simulink model "HANcoder_E407_TTA_Template_DS_V52"  (R2023a)
settings: Solver=FixedStepDiscrete  StartTime=0.0  StopTime=1  FixedStep=0.01  RelTol=1e-3
PreLoadFcn:
  | librarySetup
  | eval([bdroot,'_startup']) %Calling [modelName]_startup.m
values from neighbouring files (symbols this model uses):
  basic_cycle_duration_bc0 = TM_Reset_Board   + COMP_duration    (= 372)    [HANcoder_E407_TTA_Template_DS_V1_startup.m]    (also in HANcoder_E407_TTA_Template_DS_V2_startup.m; HANcoder_E407_TTA_Template_DS_V52_startup.m; HANcoder_E407_TTA_Template_DS_V5_startup.m; HANcoder_E407_TTA_Template_DS_V6_startup.m = 532)
  basic_cycle_duration_bc1 = basic_cycle_duration_bc0    (= 372)    [HANcoder_E407_TTA_Template_DS_V1_startup.m]    (also in HANcoder_E407_TTA_Template_DS_V2_startup.m; HANcoder_E407_TTA_Template_DS_V52_startup.m; HANcoder_E407_TTA_Template_DS_V5_startup.m; HANcoder_E407_TTA_Template_DS_V6_startup.m = 532)
  basic_cycle_duration_bc2 = basic_cycle_duration_bc0    (= 372)    [HANcoder_E407_TTA_Template_DS_V1_startup.m]    (also in HANcoder_E407_TTA_Template_DS_V2_startup.m; HANcoder_E407_TTA_Template_DS_V52_startup.m; HANcoder_E407_TTA_Template_DS_V5_startup.m; HANcoder_E407_TTA_Template_DS_V6_startup.m = 532)
  comm_delay_estimation1 = round(comm_delay_measured1*hardware_granularity/frequency_IRQ)    [HANcoder_E407_TTA_Template_DS_V1_startup.m]    (also in HANcoder_E407_TTA_Template_DS_V2_startup.m; HANcoder_E407_TTA_Template_DS_V52_startup.m; HANcoder_E407_TTA_Template_DS_V5_startup.m; HANcoder_E407_TTA_Template_DS_V6_startup.m)
  comm_delay_estimation2 = round(comm_delay_measured2*hardware_granularity/frequency_IRQ)    [HANcoder_E407_TTA_Template_DS_V1_startup.m]    (also in HANcoder_E407_TTA_Template_DS_V2_startup.m; HANcoder_E407_TTA_Template_DS_V52_startup.m; HANcoder_E407_TTA_Template_DS_V5_startup.m; HANcoder_E407_TTA_Template_DS_V6_startup.m)
  COMM_Period = 80    [HANcoder_E407_TTA_Template_DS_V1_startup.m]    (also in HANcoder_E407_TTA_Template_DS_V2_startup.m; HANcoder_E407_TTA_Template_DS_V52_startup.m; HANcoder_E407_TTA_Template_DS_V5_startup.m; HANcoder_E407_TTA_Template_DS_V6_startup.m = 120)
  COMM_Phase1 = Simulink.Parameter    [HANcoder_E407_TTA_Template_DS_V1_startup.m]    (also in HANcoder_E407_TTA_Template_DS_V2_startup.m; HANcoder_E407_TTA_Template_DS_V52_startup.m; HANcoder_E407_TTA_Template_DS_V5_startup.m; HANcoder_E407_TTA_Template_DS_V6_startup.m)
  COMM_Phase2 = Simulink.Parameter    [HANcoder_E407_TTA_Template_DS_V1_startup.m]    (also in HANcoder_E407_TTA_Template_DS_V2_startup.m; HANcoder_E407_TTA_Template_DS_V52_startup.m; HANcoder_E407_TTA_Template_DS_V5_startup.m; HANcoder_E407_TTA_Template_DS_V6_startup.m)
  COMM_Phase_init1 = Simulink.Parameter    [HANcoder_E407_TTA_Template_DS_V1_startup.m]    (also in HANcoder_E407_TTA_Template_DS_V2_startup.m; HANcoder_E407_TTA_Template_DS_V52_startup.m; HANcoder_E407_TTA_Template_DS_V5_startup.m; HANcoder_E407_TTA_Template_DS_V6_startup.m)
  COMM_Phase_init2 = Simulink.Parameter    [HANcoder_E407_TTA_Template_DS_V1_startup.m]    (also in HANcoder_E407_TTA_Template_DS_V2_startup.m; HANcoder_E407_TTA_Template_DS_V52_startup.m; HANcoder_E407_TTA_Template_DS_V5_startup.m; HANcoder_E407_TTA_Template_DS_V6_startup.m)
  COMP_duration = 4    [HANcoder_E407_TTA_Template_DS_V1_startup.m]    (also in HANcoder_E407_TTA_Template_DS_V2_startup.m; HANcoder_E407_TTA_Template_DS_V52_startup.m; HANcoder_E407_TTA_Template_DS_V5_startup.m; HANcoder_E407_TTA_Template_DS_V6_startup.m)
  frequency_IRQ = 100    [HANcoder_E407_TTA_Template_DS_V1_startup.m]    (also in HANcoder_E407_TTA_Template_DS_V2_startup.m; HANcoder_E407_TTA_Template_DS_V52_startup.m; HANcoder_E407_TTA_Template_DS_V5_startup.m; HANcoder_E407_TTA_Template_DS_V6_startup.m)
  idle_time_init = basic_cycle_duration_bc0 + basic_cycle_duration_bc1    (= 744)    [HANcoder_E407_TTA_Template_DS_V1_startup.m]    (also in HANcoder_E407_TTA_Template_DS_V2_startup.m; HANcoder_E407_TTA_Template_DS_V52_startup.m = 1116; HANcoder_E407_TTA_Template_DS_V5_startup.m = 1116; HANcoder_E407_TTA_Template_DS_V6_startup.m = 1596)
  L0b = 0.5    [HANcoder_E407_TTA_Template_DS_V52_startup.m]    (also in HANcoder_E407_TTA_Template_DS_V5_startup.m; HANcoder_E407_TTA_Template_DS_V6_startup.m)
  L0f = 5    [HANcoder_E407_TTA_Template_DS_V52_startup.m]    (also in HANcoder_E407_TTA_Template_DS_V5_startup.m; HANcoder_E407_TTA_Template_DS_V6_startup.m)
  L1f = 6    [HANcoder_E407_TTA_Template_DS_V52_startup.m]    (also in HANcoder_E407_TTA_Template_DS_V5_startup.m; HANcoder_E407_TTA_Template_DS_V6_startup.m)
  LA_Clock_Gr = 1    [HANcoder_E407_TTA_Template_DS_V1_startup.m]    (also in HANcoder_E407_TTA_Template_DS_V2_startup.m; HANcoder_E407_TTA_Template_DS_V52_startup.m; HANcoder_E407_TTA_Template_DS_V5_startup.m; HANcoder_E407_TTA_Template_DS_V6_startup.m)
  LA_COMM_dly = 1    [HANcoder_E407_TTA_Template_DS_V1_startup.m]    (also in HANcoder_E407_TTA_Template_DS_V2_startup.m; HANcoder_E407_TTA_Template_DS_V52_startup.m; HANcoder_E407_TTA_Template_DS_V5_startup.m; HANcoder_E407_TTA_Template_DS_V6_startup.m)
  LA_COMM_Err = 1    [HANcoder_E407_TTA_Template_DS_V1_startup.m]    (also in HANcoder_E407_TTA_Template_DS_V2_startup.m; HANcoder_E407_TTA_Template_DS_V52_startup.m; HANcoder_E407_TTA_Template_DS_V5_startup.m; HANcoder_E407_TTA_Template_DS_V6_startup.m)
  LA_E_Desync = 1    [HANcoder_E407_TTA_Template_DS_V1_startup.m]    (also in HANcoder_E407_TTA_Template_DS_V2_startup.m; HANcoder_E407_TTA_Template_DS_V52_startup.m; HANcoder_E407_TTA_Template_DS_V5_startup.m; HANcoder_E407_TTA_Template_DS_V6_startup.m)
  LA_MEX_Flag = 1    [HANcoder_E407_TTA_Template_DS_V1_startup.m]    (also in HANcoder_E407_TTA_Template_DS_V2_startup.m; HANcoder_E407_TTA_Template_DS_V52_startup.m; HANcoder_E407_TTA_Template_DS_V5_startup.m; HANcoder_E407_TTA_Template_DS_V6_startup.m)
  LA_Task_Act = 1    [HANcoder_E407_TTA_Template_DS_V1_startup.m]    (also in HANcoder_E407_TTA_Template_DS_V2_startup.m; HANcoder_E407_TTA_Template_DS_V52_startup.m; HANcoder_E407_TTA_Template_DS_V5_startup.m; HANcoder_E407_TTA_Template_DS_V6_startup.m)
  Master_Role = 1    [HANcoder_E407_TTA_Template_DS_V1_startup.m]    (also in HANcoder_E407_TTA_Template_DS_V2_startup.m; HANcoder_E407_TTA_Template_DS_V52_startup.m; HANcoder_E407_TTA_Template_DS_V5_startup.m; HANcoder_E407_TTA_Template_DS_V6_startup.m)
  matrix_rows = 3    [HANcoder_E407_TTA_Template_DS_V1_startup.m]    (also in HANcoder_E407_TTA_Template_DS_V2_startup.m; HANcoder_E407_TTA_Template_DS_V52_startup.m; HANcoder_E407_TTA_Template_DS_V5_startup.m; HANcoder_E407_TTA_Template_DS_V6_startup.m)
  max_desync = 15    [HANcoder_E407_TTA_Template_DS_V1_startup.m]    (also in HANcoder_E407_TTA_Template_DS_V2_startup.m; HANcoder_E407_TTA_Template_DS_V52_startup.m; HANcoder_E407_TTA_Template_DS_V5_startup.m; HANcoder_E407_TTA_Template_DS_V6_startup.m)
  max_num_msgs_CAN1 = 2^Tx_bit_number-1    (= 7)    [HANcoder_E407_TTA_Template_DS_V1_startup.m]    (also in HANcoder_E407_TTA_Template_DS_V2_startup.m; HANcoder_E407_TTA_Template_DS_V52_startup.m; HANcoder_E407_TTA_Template_DS_V5_startup.m; HANcoder_E407_TTA_Template_DS_V6_startup.m)
  max_num_msgs_CAN2 = max_num_msgs_CAN1    (= 7)    [HANcoder_E407_TTA_Template_DS_V1_startup.m]    (also in HANcoder_E407_TTA_Template_DS_V2_startup.m; HANcoder_E407_TTA_Template_DS_V52_startup.m; HANcoder_E407_TTA_Template_DS_V5_startup.m; HANcoder_E407_TTA_Template_DS_V6_startup.m)
  min_desync = (-1)*max_desync    (= -15)    [HANcoder_E407_TTA_Template_DS_V1_startup.m]    (also in HANcoder_E407_TTA_Template_DS_V2_startup.m; HANcoder_E407_TTA_Template_DS_V52_startup.m; HANcoder_E407_TTA_Template_DS_V5_startup.m; HANcoder_E407_TTA_Template_DS_V6_startup.m)
  PID_derivative = Simulink.Parameter    [HANcoder_E407_TTA_Template_DS_V52_startup.m]    (also in HANcoder_E407_TTA_Template_DS_V6_startup.m)
  PID_gain = Simulink.Parameter    [HANcoder_E407_TTA_Template_DS_V52_startup.m]    (also in HANcoder_E407_TTA_Template_DS_V6_startup.m)
  PID_integrator = Simulink.Parameter    [HANcoder_E407_TTA_Template_DS_V52_startup.m]    (also in HANcoder_E407_TTA_Template_DS_V6_startup.m)
  PotValue1_ID = 22    [HANcoder_E407_TTA_Template_DS_V1_startup.m]    (also in HANcoder_E407_TTA_Template_DS_V2_startup.m; HANcoder_E407_TTA_Template_DS_V52_startup.m; HANcoder_E407_TTA_Template_DS_V5_startup.m; HANcoder_E407_TTA_Template_DS_V6_startup.m)
  PotValue2_ID = 23    [HANcoder_E407_TTA_Template_DS_V1_startup.m]    (also in HANcoder_E407_TTA_Template_DS_V2_startup.m; HANcoder_E407_TTA_Template_DS_V52_startup.m; HANcoder_E407_TTA_Template_DS_V5_startup.m; HANcoder_E407_TTA_Template_DS_V6_startup.m)
  PotValue3_ID = 24    [HANcoder_E407_TTA_Template_DS_V1_startup.m]    (also in HANcoder_E407_TTA_Template_DS_V2_startup.m; HANcoder_E407_TTA_Template_DS_V52_startup.m; HANcoder_E407_TTA_Template_DS_V5_startup.m; HANcoder_E407_TTA_Template_DS_V6_startup.m)
  script_run = Simulink.Parameter    [HANcoder_E407_TTA_Template_DS_V1_startup.m]    (also in HANcoder_E407_TTA_Template_DS_V2_startup.m; HANcoder_E407_TTA_Template_DS_V52_startup.m; HANcoder_E407_TTA_Template_DS_V5_startup.m; HANcoder_E407_TTA_Template_DS_V6_startup.m)
  Slave_Role = 2    [HANcoder_E407_TTA_Template_DS_V1_startup.m]    (also in HANcoder_E407_TTA_Template_DS_V2_startup.m; HANcoder_E407_TTA_Template_DS_V52_startup.m; HANcoder_E407_TTA_Template_DS_V5_startup.m; HANcoder_E407_TTA_Template_DS_V6_startup.m)
  Sync_ID = 1    [HANcoder_E407_TTA_Template_DS_V1_startup.m]    (also in HANcoder_E407_TTA_Template_DS_V2_startup.m; HANcoder_E407_TTA_Template_DS_V52_startup.m; HANcoder_E407_TTA_Template_DS_V5_startup.m; HANcoder_E407_TTA_Template_DS_V6_startup.m)
  TM_Check_PotValue1 = TM_COMM_PotValue1 + COMM_duration    (= 174)    [HANcoder_E407_TTA_Template_DS_V1_startup.m]    (also in HANcoder_E407_TTA_Template_DS_V2_startup.m; HANcoder_E407_TTA_Template_DS_V52_startup.m; HANcoder_E407_TTA_Template_DS_V5_startup.m; HANcoder_E407_TTA_Template_DS_V6_startup.m = 254)
  TM_Check_PotValue2 = TM_COMM_PotValue2 + COMM_duration    (= 258)    [HANcoder_E407_TTA_Template_DS_V1_startup.m]    (also in HANcoder_E407_TTA_Template_DS_V2_startup.m; HANcoder_E407_TTA_Template_DS_V52_startup.m; HANcoder_E407_TTA_Template_DS_V5_startup.m; HANcoder_E407_TTA_Template_DS_V6_startup.m = 378)
  TM_Check_PotValue3 = TM_COMM_PotValue3 + COMM_duration    (= 342)    [HANcoder_E407_TTA_Template_DS_V1_startup.m]    (also in HANcoder_E407_TTA_Template_DS_V2_startup.m; HANcoder_E407_TTA_Template_DS_V52_startup.m; HANcoder_E407_TTA_Template_DS_V5_startup.m; HANcoder_E407_TTA_Template_DS_V6_startup.m = 502)
  TM_Check_Sync = TM_COMM_Sync   + COMM_duration    (= 80)    [HANcoder_E407_TTA_Template_DS_V1_startup.m]    (also in HANcoder_E407_TTA_Template_DS_V2_startup.m; HANcoder_E407_TTA_Template_DS_V52_startup.m; HANcoder_E407_TTA_Template_DS_V5_startup.m; HANcoder_E407_TTA_Template_DS_V6_startup.m = 120)
  TM_Check_TOuts = TM_Count_Vote3 + COMP_duration    (= 356)    [HANcoder_E407_TTA_Template_DS_V1_startup.m]    (also in HANcoder_E407_TTA_Template_DS_V2_startup.m; HANcoder_E407_TTA_Template_DS_V52_startup.m; HANcoder_E407_TTA_Template_DS_V5_startup.m; HANcoder_E407_TTA_Template_DS_V6_startup.m = 516)
  TM_Check_Trailer1Articulation = TM_COMM_Trailer1Articulation + COMM_duration    (= 170)    [HANcoder_E407_TTA_Template_DS_V1_startup.m]    (also in HANcoder_E407_TTA_Template_DS_V2_startup.m; HANcoder_E407_TTA_Template_DS_V52_startup.m; HANcoder_E407_TTA_Template_DS_V5_startup.m; HANcoder_E407_TTA_Template_DS_V6_startup.m = 250)
  TM_Check_Trailer2Articulation = TM_COMM_Trailer2Articulation + COMM_duration    (= 254)    [HANcoder_E407_TTA_Template_DS_V1_startup.m]    (also in HANcoder_E407_TTA_Template_DS_V2_startup.m; HANcoder_E407_TTA_Template_DS_V52_startup.m; HANcoder_E407_TTA_Template_DS_V5_startup.m; HANcoder_E407_TTA_Template_DS_V6_startup.m = 374)
  TM_Check_Vote1 = TM_COMM_Vote1  + COMM_duration    (= 172)    [HANcoder_E407_TTA_Template_DS_V1_startup.m]    (also in HANcoder_E407_TTA_Template_DS_V2_startup.m; HANcoder_E407_TTA_Template_DS_V52_startup.m; HANcoder_E407_TTA_Template_DS_V5_startup.m; HANcoder_E407_TTA_Template_DS_V6_startup.m = 252)
  TM_Check_Vote2 = TM_COMM_Vote2  + COMM_duration    (= 260)    [HANcoder_E407_TTA_Template_DS_V1_startup.m]    (also in HANcoder_E407_TTA_Template_DS_V2_startup.m; HANcoder_E407_TTA_Template_DS_V52_startup.m; HANcoder_E407_TTA_Template_DS_V5_startup.m; HANcoder_E407_TTA_Template_DS_V6_startup.m = 380)
  TM_Check_Vote3 = TM_COMM_Vote3  + COMM_duration    (= 348)    [HANcoder_E407_TTA_Template_DS_V1_startup.m]    (also in HANcoder_E407_TTA_Template_DS_V2_startup.m; HANcoder_E407_TTA_Template_DS_V52_startup.m; HANcoder_E407_TTA_Template_DS_V5_startup.m; HANcoder_E407_TTA_Template_DS_V6_startup.m = 508)
  TM_COMM_PotValue1 = TM_ReadPot + COMP_duration    (= 94)    [HANcoder_E407_TTA_Template_DS_V1_startup.m]    (also in HANcoder_E407_TTA_Template_DS_V2_startup.m; HANcoder_E407_TTA_Template_DS_V52_startup.m; HANcoder_E407_TTA_Template_DS_V5_startup.m; HANcoder_E407_TTA_Template_DS_V6_startup.m = 134)
  TM_COMM_PotValue2 = TM_Check_PotValue1 + COMP_duration    (= 178)    [HANcoder_E407_TTA_Template_DS_V1_startup.m]    (also in HANcoder_E407_TTA_Template_DS_V2_startup.m; HANcoder_E407_TTA_Template_DS_V52_startup.m; HANcoder_E407_TTA_Template_DS_V5_startup.m; HANcoder_E407_TTA_Template_DS_V6_startup.m = 258)
  TM_COMM_PotValue3 = TM_Check_PotValue2 + COMP_duration    (= 262)    [HANcoder_E407_TTA_Template_DS_V1_startup.m]    (also in HANcoder_E407_TTA_Template_DS_V2_startup.m; HANcoder_E407_TTA_Template_DS_V52_startup.m; HANcoder_E407_TTA_Template_DS_V5_startup.m; HANcoder_E407_TTA_Template_DS_V6_startup.m = 382)
  TM_COMM_Sync = basic_cycle_start    (= 0)    [HANcoder_E407_TTA_Template_DS_V1_startup.m]    (also in HANcoder_E407_TTA_Template_DS_V2_startup.m; HANcoder_E407_TTA_Template_DS_V52_startup.m; HANcoder_E407_TTA_Template_DS_V5_startup.m; HANcoder_E407_TTA_Template_DS_V6_startup.m)
  TM_COMM_Trailer1Articulation = TM_Update_LT_2 + COMP_duration    (= 90)    [HANcoder_E407_TTA_Template_DS_V1_startup.m]    (also in HANcoder_E407_TTA_Template_DS_V2_startup.m; HANcoder_E407_TTA_Template_DS_V52_startup.m; HANcoder_E407_TTA_Template_DS_V5_startup.m; HANcoder_E407_TTA_Template_DS_V6_startup.m = 130)
  TM_COMM_Trailer2Articulation = TM_Check_Trailer1Articulation + COMP_duration    (= 174)    [HANcoder_E407_TTA_Template_DS_V1_startup.m]    (also in HANcoder_E407_TTA_Template_DS_V2_startup.m; HANcoder_E407_TTA_Template_DS_V52_startup.m; HANcoder_E407_TTA_Template_DS_V5_startup.m; HANcoder_E407_TTA_Template_DS_V6_startup.m = 254)
  TM_COMM_Vote1 = TM_Vote_Dec    + COMP_duration    (= 92)    [HANcoder_E407_TTA_Template_DS_V1_startup.m]    (also in HANcoder_E407_TTA_Template_DS_V2_startup.m; HANcoder_E407_TTA_Template_DS_V52_startup.m; HANcoder_E407_TTA_Template_DS_V5_startup.m; HANcoder_E407_TTA_Template_DS_V6_startup.m = 132)
  TM_COMM_Vote2 = TM_Count_Vote1 + COMP_duration    (= 180)    [HANcoder_E407_TTA_Template_DS_V1_startup.m]    (also in HANcoder_E407_TTA_Template_DS_V2_startup.m; HANcoder_E407_TTA_Template_DS_V52_startup.m; HANcoder_E407_TTA_Template_DS_V5_startup.m; HANcoder_E407_TTA_Template_DS_V6_startup.m = 260)
  TM_COMM_Vote3 = TM_Count_Vote2 + COMP_duration    (= 268)    [HANcoder_E407_TTA_Template_DS_V1_startup.m]    (also in HANcoder_E407_TTA_Template_DS_V2_startup.m; HANcoder_E407_TTA_Template_DS_V52_startup.m; HANcoder_E407_TTA_Template_DS_V5_startup.m; HANcoder_E407_TTA_Template_DS_V6_startup.m = 388)
  TM_Count_Vote1 = TM_Check_Vote1 + COMP_duration    (= 176)    [HANcoder_E407_TTA_Template_DS_V1_startup.m]    (also in HANcoder_E407_TTA_Template_DS_V2_startup.m; HANcoder_E407_TTA_Template_DS_V52_startup.m; HANcoder_E407_TTA_Template_DS_V5_startup.m; HANcoder_E407_TTA_Template_DS_V6_startup.m = 256)
  TM_Count_Vote2 = TM_Check_Vote2 + COMP_duration    (= 264)    [HANcoder_E407_TTA_Template_DS_V1_startup.m]    (also in HANcoder_E407_TTA_Template_DS_V2_startup.m; HANcoder_E407_TTA_Template_DS_V52_startup.m; HANcoder_E407_TTA_Template_DS_V5_startup.m; HANcoder_E407_TTA_Template_DS_V6_startup.m = 384)
  TM_Count_Vote3 = TM_Check_Vote3 + COMP_duration    (= 352)    [HANcoder_E407_TTA_Template_DS_V1_startup.m]    (also in HANcoder_E407_TTA_Template_DS_V2_startup.m; HANcoder_E407_TTA_Template_DS_V52_startup.m; HANcoder_E407_TTA_Template_DS_V5_startup.m; HANcoder_E407_TTA_Template_DS_V6_startup.m = 512)
  TM_Data_bc0 = TM_COMM_Sync    (= 0)    [HANcoder_E407_TTA_Template_DS_V1_startup.m]    (also in HANcoder_E407_TTA_Template_DS_V2_startup.m; HANcoder_E407_TTA_Template_DS_V52_startup.m; HANcoder_E407_TTA_Template_DS_V5_startup.m; HANcoder_E407_TTA_Template_DS_V6_startup.m)
  TM_Data_bc1 = TM_Data_bc0(1:4)    [HANcoder_E407_TTA_Template_DS_V1_startup.m]    (also in HANcoder_E407_TTA_Template_DS_V2_startup.m; HANcoder_E407_TTA_Template_DS_V52_startup.m; HANcoder_E407_TTA_Template_DS_V5_startup.m; HANcoder_E407_TTA_Template_DS_V6_startup.m)
  TM_Data_bc2 = TM_Data_bc0(1:4)    [HANcoder_E407_TTA_Template_DS_V1_startup.m]    (also in HANcoder_E407_TTA_Template_DS_V2_startup.m; HANcoder_E407_TTA_Template_DS_V52_startup.m; HANcoder_E407_TTA_Template_DS_V5_startup.m; HANcoder_E407_TTA_Template_DS_V6_startup.m)
  TM_InverseKinematics = TM_Check_Trailer2Articulation + COMP_duration    (= 258)    [HANcoder_E407_TTA_Template_DS_V1_startup.m]    (also in HANcoder_E407_TTA_Template_DS_V2_startup.m; HANcoder_E407_TTA_Template_DS_V52_startup.m; HANcoder_E407_TTA_Template_DS_V5_startup.m; HANcoder_E407_TTA_Template_DS_V6_startup.m = 378)
  TM_New_Master = TM_Check_TOuts + COMP_duration    (= 360)    [HANcoder_E407_TTA_Template_DS_V1_startup.m]    (also in HANcoder_E407_TTA_Template_DS_V2_startup.m; HANcoder_E407_TTA_Template_DS_V52_startup.m; HANcoder_E407_TTA_Template_DS_V5_startup.m; HANcoder_E407_TTA_Template_DS_V6_startup.m = 520)
  TM_PotVote = TM_COMM_PotValue3 + COMP_duration    (= 266)    [HANcoder_E407_TTA_Template_DS_V1_startup.m]    (also in HANcoder_E407_TTA_Template_DS_V2_startup.m; HANcoder_E407_TTA_Template_DS_V52_startup.m; HANcoder_E407_TTA_Template_DS_V5_startup.m; HANcoder_E407_TTA_Template_DS_V6_startup.m = 386)
  TM_ReadPot = TM_Update_LT_2 + COMP_duration    (= 90)    [HANcoder_E407_TTA_Template_DS_V1_startup.m]    (also in HANcoder_E407_TTA_Template_DS_V2_startup.m; HANcoder_E407_TTA_Template_DS_V52_startup.m; HANcoder_E407_TTA_Template_DS_V5_startup.m; HANcoder_E407_TTA_Template_DS_V6_startup.m = 130)
  TM_Reset_Board = TM_Reset_Var   + COMP_duration    (= 368)    [HANcoder_E407_TTA_Template_DS_V1_startup.m]    (also in HANcoder_E407_TTA_Template_DS_V2_startup.m; HANcoder_E407_TTA_Template_DS_V52_startup.m; HANcoder_E407_TTA_Template_DS_V5_startup.m; HANcoder_E407_TTA_Template_DS_V6_startup.m = 528)
  TM_Reset_Var = TM_New_Master  + COMP_duration    (= 364)    [HANcoder_E407_TTA_Template_DS_V1_startup.m]    (also in HANcoder_E407_TTA_Template_DS_V2_startup.m; HANcoder_E407_TTA_Template_DS_V52_startup.m; HANcoder_E407_TTA_Template_DS_V5_startup.m; HANcoder_E407_TTA_Template_DS_V6_startup.m = 524)
  TM_Reset_Var_bc1 = TM_Data_bc1(end) + COMP_duration    [HANcoder_E407_TTA_Template_DS_V1_startup.m]    (also in HANcoder_E407_TTA_Template_DS_V2_startup.m; HANcoder_E407_TTA_Template_DS_V52_startup.m; HANcoder_E407_TTA_Template_DS_V5_startup.m; HANcoder_E407_TTA_Template_DS_V6_startup.m)
  TM_Reset_Var_bc1_2 = TM_Reset_Var_bc1 +2    [HANcoder_E407_TTA_Template_DS_V1_startup.m]    (also in HANcoder_E407_TTA_Template_DS_V2_startup.m; HANcoder_E407_TTA_Template_DS_V52_startup.m; HANcoder_E407_TTA_Template_DS_V5_startup.m; HANcoder_E407_TTA_Template_DS_V6_startup.m)
  TM_Reset_Var_bc2 = TM_Data_bc2(end) + COMP_duration    [HANcoder_E407_TTA_Template_DS_V1_startup.m]    (also in HANcoder_E407_TTA_Template_DS_V2_startup.m; HANcoder_E407_TTA_Template_DS_V52_startup.m; HANcoder_E407_TTA_Template_DS_V5_startup.m; HANcoder_E407_TTA_Template_DS_V6_startup.m)
  TM_Reset_Var_bc2_2 = TM_Reset_Var_bc2 +2    [HANcoder_E407_TTA_Template_DS_V1_startup.m]    (also in HANcoder_E407_TTA_Template_DS_V2_startup.m; HANcoder_E407_TTA_Template_DS_V52_startup.m; HANcoder_E407_TTA_Template_DS_V5_startup.m; HANcoder_E407_TTA_Template_DS_V6_startup.m)
  TM_SteerControl = TM_InverseKinematics + COMP_duration    (= 262)    [HANcoder_E407_TTA_Template_DS_V1_startup.m]    (also in HANcoder_E407_TTA_Template_DS_V2_startup.m; HANcoder_E407_TTA_Template_DS_V52_startup.m = 259; HANcoder_E407_TTA_Template_DS_V5_startup.m = 259)
  TM_Type_bc0 = COMM    (= 0)    [HANcoder_E407_TTA_Template_DS_V1_startup.m]    (also in HANcoder_E407_TTA_Template_DS_V2_startup.m; HANcoder_E407_TTA_Template_DS_V52_startup.m; HANcoder_E407_TTA_Template_DS_V5_startup.m; HANcoder_E407_TTA_Template_DS_V6_startup.m)
  TM_Type_bc1 = TM_Type_bc0(1:4)    [HANcoder_E407_TTA_Template_DS_V1_startup.m]    (also in HANcoder_E407_TTA_Template_DS_V2_startup.m; HANcoder_E407_TTA_Template_DS_V52_startup.m; HANcoder_E407_TTA_Template_DS_V5_startup.m; HANcoder_E407_TTA_Template_DS_V6_startup.m)
  TM_Type_bc2 = TM_Type_bc0(1:4)    [HANcoder_E407_TTA_Template_DS_V1_startup.m]    (also in HANcoder_E407_TTA_Template_DS_V2_startup.m; HANcoder_E407_TTA_Template_DS_V52_startup.m; HANcoder_E407_TTA_Template_DS_V5_startup.m; HANcoder_E407_TTA_Template_DS_V6_startup.m)
  TM_Update_LT = TM_Check_Sync  + COMP_duration    (= 84)    [HANcoder_E407_TTA_Template_DS_V1_startup.m]    (also in HANcoder_E407_TTA_Template_DS_V2_startup.m; HANcoder_E407_TTA_Template_DS_V52_startup.m; HANcoder_E407_TTA_Template_DS_V5_startup.m; HANcoder_E407_TTA_Template_DS_V6_startup.m = 124)
  TM_Update_LT_2 = TM_Update_LT   + 2    (= 86)    [HANcoder_E407_TTA_Template_DS_V1_startup.m]    (also in HANcoder_E407_TTA_Template_DS_V2_startup.m; HANcoder_E407_TTA_Template_DS_V52_startup.m; HANcoder_E407_TTA_Template_DS_V5_startup.m; HANcoder_E407_TTA_Template_DS_V6_startup.m = 126)
  TM_Vote_Dec = TM_Update_LT   + COMP_duration    (= 88)    [HANcoder_E407_TTA_Template_DS_V1_startup.m]    (also in HANcoder_E407_TTA_Template_DS_V2_startup.m; HANcoder_E407_TTA_Template_DS_V52_startup.m; HANcoder_E407_TTA_Template_DS_V5_startup.m; HANcoder_E407_TTA_Template_DS_V6_startup.m = 128)
  Tractor_Board1 = 11    [HANcoder_E407_TTA_Template_DS_V1_startup.m]    (also in HANcoder_E407_TTA_Template_DS_V2_startup.m = 1; HANcoder_E407_TTA_Template_DS_V52_startup.m = 1; HANcoder_E407_TTA_Template_DS_V5_startup.m = 1; HANcoder_E407_TTA_Template_DS_V6_startup.m = 1)
  Tractor_Board2 = 12    [HANcoder_E407_TTA_Template_DS_V1_startup.m]    (also in HANcoder_E407_TTA_Template_DS_V2_startup.m = 2; HANcoder_E407_TTA_Template_DS_V52_startup.m = 2; HANcoder_E407_TTA_Template_DS_V5_startup.m = 2; HANcoder_E407_TTA_Template_DS_V6_startup.m = 2)
  Tractor_Board3 = 13    [HANcoder_E407_TTA_Template_DS_V1_startup.m]    (also in HANcoder_E407_TTA_Template_DS_V2_startup.m = 3; HANcoder_E407_TTA_Template_DS_V52_startup.m = 3; HANcoder_E407_TTA_Template_DS_V5_startup.m = 3; HANcoder_E407_TTA_Template_DS_V6_startup.m = 3)
  Trailer1_Articulation_ID = 31    [HANcoder_E407_TTA_Template_DS_V1_startup.m]    (also in HANcoder_E407_TTA_Template_DS_V2_startup.m; HANcoder_E407_TTA_Template_DS_V52_startup.m; HANcoder_E407_TTA_Template_DS_V5_startup.m; HANcoder_E407_TTA_Template_DS_V6_startup.m)
  Trailer1_Board1 = 2    [HANcoder_E407_TTA_Template_DS_V1_startup.m]    (also in HANcoder_E407_TTA_Template_DS_V2_startup.m = 4; HANcoder_E407_TTA_Template_DS_V52_startup.m = 4; HANcoder_E407_TTA_Template_DS_V5_startup.m = 4; HANcoder_E407_TTA_Template_DS_V6_startup.m = 4)
  Trailer1_Board2 = 3    [HANcoder_E407_TTA_Template_DS_V1_startup.m]    (also in HANcoder_E407_TTA_Template_DS_V2_startup.m = 5; HANcoder_E407_TTA_Template_DS_V52_startup.m = 5; HANcoder_E407_TTA_Template_DS_V5_startup.m = 5; HANcoder_E407_TTA_Template_DS_V6_startup.m = 5)
  Trailer1_Board3 = 4    [HANcoder_E407_TTA_Template_DS_V1_startup.m]    (also in HANcoder_E407_TTA_Template_DS_V2_startup.m = 6; HANcoder_E407_TTA_Template_DS_V52_startup.m = 6; HANcoder_E407_TTA_Template_DS_V5_startup.m = 6; HANcoder_E407_TTA_Template_DS_V6_startup.m = 6)
  Trailer2_Articulation_ID = 32    [HANcoder_E407_TTA_Template_DS_V1_startup.m]    (also in HANcoder_E407_TTA_Template_DS_V2_startup.m; HANcoder_E407_TTA_Template_DS_V52_startup.m; HANcoder_E407_TTA_Template_DS_V5_startup.m; HANcoder_E407_TTA_Template_DS_V6_startup.m)
  Trailer2_Board1 = 5    [HANcoder_E407_TTA_Template_DS_V1_startup.m]    (also in HANcoder_E407_TTA_Template_DS_V2_startup.m = 7; HANcoder_E407_TTA_Template_DS_V52_startup.m = 7; HANcoder_E407_TTA_Template_DS_V5_startup.m = 7; HANcoder_E407_TTA_Template_DS_V6_startup.m = 7)
  Trailer2_Board2 = 6    [HANcoder_E407_TTA_Template_DS_V1_startup.m]    (also in HANcoder_E407_TTA_Template_DS_V2_startup.m = 8; HANcoder_E407_TTA_Template_DS_V52_startup.m = 8; HANcoder_E407_TTA_Template_DS_V5_startup.m = 8; HANcoder_E407_TTA_Template_DS_V6_startup.m = 8)
  Trailer2_Board3 = 7    [HANcoder_E407_TTA_Template_DS_V1_startup.m]    (also in HANcoder_E407_TTA_Template_DS_V2_startup.m = 9; HANcoder_E407_TTA_Template_DS_V52_startup.m = 9; HANcoder_E407_TTA_Template_DS_V5_startup.m = 9; HANcoder_E407_TTA_Template_DS_V6_startup.m = 9)
  V1 = -0.000000001    (= -1e-09)    [HANcoder_E407_TTA_Template_DS_V52_startup.m]    (also in HANcoder_E407_TTA_Template_DS_V5_startup.m; HANcoder_E407_TTA_Template_DS_V6_startup.m)
  V2 = -0.000000001    (= -1e-09)    [HANcoder_E407_TTA_Template_DS_V52_startup.m]    (also in HANcoder_E407_TTA_Template_DS_V5_startup.m; HANcoder_E407_TTA_Template_DS_V6_startup.m)
  Vote1_ID = 11    [HANcoder_E407_TTA_Template_DS_V1_startup.m]    (also in HANcoder_E407_TTA_Template_DS_V2_startup.m; HANcoder_E407_TTA_Template_DS_V52_startup.m; HANcoder_E407_TTA_Template_DS_V5_startup.m; HANcoder_E407_TTA_Template_DS_V6_startup.m)
  Vote2_ID = 12    [HANcoder_E407_TTA_Template_DS_V1_startup.m]    (also in HANcoder_E407_TTA_Template_DS_V2_startup.m; HANcoder_E407_TTA_Template_DS_V52_startup.m; HANcoder_E407_TTA_Template_DS_V5_startup.m; HANcoder_E407_TTA_Template_DS_V6_startup.m)
  Vote3_ID = 13    [HANcoder_E407_TTA_Template_DS_V1_startup.m]    (also in HANcoder_E407_TTA_Template_DS_V2_startup.m; HANcoder_E407_TTA_Template_DS_V52_startup.m; HANcoder_E407_TTA_Template_DS_V5_startup.m; HANcoder_E407_TTA_Template_DS_V6_startup.m)
undefined symbols (not defined in the file or in its folder): A0, A1, A2, A3, A4, A5, CON2, CON3, CON4, D10, D12, D13, D6, D7, D8, D9
libraries: hdlsllib x136, simulink x39, HANcoder_STM32_Target x31, simulink_extras x8, dspstat3 x2, slpidlib x1
(part 24 of 40)

== system HANcoder_E407_TTA_Template_DS_V52/HANcoder STM32 Target - E407-STM32 algorithm/TTA CAN System/TTA System/Matrix Cycle Manager/Controller Matrix Cycle/controller basic cycle 1/COMP Task - Sync bc1 check/Process_Messages ==
  note: Logic Analyzer - DEBUG
      | Sync_Check COMP task
      | activation
  note: Logic Analyzer - DEBUG
  new_CAN1_msg : Inport
  new_CAN2_msg : Inport  Port=2
  Rx_msg_CAN1 : Inport  Port=3  OutDataTypeStr=Bus: msg_buffer_type
  Rx_Msg_CAN2 : Inport  Port=4  OutDataTypeStr=Bus: msg_buffer_type
  expected_basic_cycle : Inport  Port=5
  TM_COMM : Inport  Port=6
  expected_board_id : Inport  Port=7
  Enable : EnablePort
  Bus Selector : BusSelector  OutputSignals=signal1,Buffer_2,Buffer_3,Buffer_4,Buffer_5,Buffer_6,Buffer_7,Buffer_8
  Constant2 : Constant  Priority=28  OutDataTypeStr=boolean
  Data Store Write : DataStoreWrite  Priority=4  DataStoreName=Msg_Rx  DataStoreElements=Msg_Rx.Buffer_1#Msg_Rx.Buffer_2#Msg_Rx.Buffer_3#Msg_Rx.Buffer_4#Msg_Rx.Buffer_5#Msg_Rx.Buffer_6#Msg_Rx.Buffer_7#Msg_Rx.Buffer_8  IndexOptions=Index vector (dialog)  Indices=1  OutputSizes=1
  Data Store Write2 : DataStoreWrite  DataStoreName=new_msg_Rx  IndexOptions=Index vector (dialog)  Indices=1  OutputSizes=1
  Data Store Write3 : DataStoreWrite  Priority=29  DataStoreName=Toggle_Pin_A0  IndexOptions=Index vector (dialog)  Indices=1  OutputSizes=1
  Demux message CAN1 and check coherence : Subsystem  Priority=1
  Demux message CAN1 and check coherence1 : Subsystem  Priority=2
  Desync calculation : Subsystem  Priority=10
  OR : Logic  Operator=OR  IconShape=distinctive  AllPortsSameDT=off  OutDataTypeStr=boolean
  Switch : Switch  Priority=3  Criteria=u2 > Threshold  SaturateOnIntegerOverflow=off  InputSameDT=off
  wires:
  new_CAN1_msg/1 -> Demux message CAN1 and check coherence/Enable
  new_CAN2_msg/1 -> Demux message CAN1 and check coherence1/Enable
  Rx_msg_CAN1/1 -> Demux message CAN1 and check coherence/1(CAN1_Rx_msg)
  Rx_Msg_CAN2/1 -> Demux message CAN1 and check coherence1/1(CAN2_Rx_msg)
  Demux message CAN1 and check coherence/1(CAN1_msg) -> Switch/1
  Demux message CAN1 and check coherence1/1(CAN2_msg_coherent) -> OR/2
  Demux message CAN1 and check coherence1/3(CAN2_msg) -> Switch/3
  expected_basic_cycle/1 -> Demux message CAN1 and check coherence1/2(expected_basic_cycle), Demux message CAN1 and check coherence/2(expected_basic_cycle)
  Constant2/1 -> Data Store Write3/1
  expected_board_id/1 -> Demux message CAN1 and check coherence1/3(expected_board_id), Demux message CAN1 and check coherence/3(expected_board_id)
  Demux message CAN1 and check coherence/2(Msg_Count_CAN1) -> [msg_count_CAN1]
  Demux message CAN1 and check coherence1/2(Msg_Count_CAN2) -> [msg_count_CAN2]
  Switch/1 -> Bus Selector/1
  Bus Selector/1 -> Data Store Write/1  "<signal1>"
  Bus Selector/2 -> Data Store Write/2  "<Buffer_2>"
  Bus Selector/3 -> Data Store Write/3  "<Buffer_3>"
  Bus Selector/4 -> Data Store Write/4  "<Buffer_4>"
  Bus Selector/5 -> Data Store Write/5  "<Buffer_5>"
  Bus Selector/6 -> Data Store Write/6  "<Buffer_6>"
  Bus Selector/7 -> Data Store Write/7  "<Buffer_7>"
  Bus Selector/8 -> Data Store Write/8  "<Buffer_8>"
  [CAN1_msg_coherent_TAG] -> Desync calculation/2(New_msg_CAN1)
  Demux message CAN1 and check coherence/3(CAN1_msg_coherent) -> [CAN1_msg_coherent_TAG], Switch/2, OR/1
  [new_msg_Rx_TAG] -> Desync calculation/Enable
  OR/1 -> [new_msg_Rx_TAG], Data Store Write2/1
  TM_COMM/1 -> Desync calculation/1(TM_COMM)
  [msg_count_CAN1] -> Desync calculation/3(msg_count_CAN1)
  [msg_count_CAN2] -> Desync calculation/4(msg_count_CAN2)

== system HANcoder_E407_TTA_Template_DS_V52/HANcoder STM32 Target - E407-STM32 algorithm/TTA CAN System/TTA System/Matrix Cycle Manager/Controller Matrix Cycle/controller basic cycle 1/COMP Task - Sync bc1 check/Reset Tx msg counter ==
  Enable : EnablePort
  Constant1 : Constant  Priority=2
  Constant6 : Constant  Priority=2
  Data Store Write1 : DataStoreWrite  Priority=4  DataStoreName=Tx_msg_count_CAN1  IndexOptions=Index vector (dialog)  Indices=1  OutputSizes=1
  Data Store Write2 : DataStoreWrite  Priority=4  DataStoreName=Tx_msg_count_CAN2  IndexOptions=Index vector (dialog)  Indices=1  OutputSizes=1
  wires:
  Constant6/1 -> Data Store Write1/1
  Constant1/1 -> Data Store Write2/1

== system HANcoder_E407_TTA_Template_DS_V52/HANcoder STM32 Target - E407-STM32 algorithm/TTA CAN System/TTA System/Matrix Cycle Manager/Controller Matrix Cycle/controller basic cycle 1/COMP Task - Update LT1/LA - Ensemble precision ==
  note: Logic Analyzer - DEBUG
      | Ensemble precision
      | measurement (Desync)
  Enable : EnablePort
  Constant2 : Constant  Priority=28  OutDataTypeStr=boolean
  Data Store Write1 : DataStoreWrite  Priority=29  DataStoreName=Toggle_Pin_D10  IndexOptions=Index vector (dialog)  Indices=1  OutputSizes=1
  wires:
  Constant2/1 -> Data Store Write1/1

== system HANcoder_E407_TTA_Template_DS_V52/HANcoder STM32 Target - E407-STM32 algorithm/TTA CAN System/TTA System/Matrix Cycle Manager/Controller Matrix Cycle/controller basic cycle 1/COMP Task - Update LT1/Local Time Update ==
  note: If the desync is negative, the Local Time
      | gets updated straight away. Otherwise,
      | the Local Time must be updated in small
      | steps.
  note: Desync Check
  note: Local Time Update Acknowledge
  note: Global - Local time update acknowledge
  note: Logic Analyzer - DEBUG
      | LT Update COMP task
      | activation
  note: Logic Analyzer - DEBUG
  note: Logic Analyzer - DEBUG
      | Ensemble precision
      | measurement (Desync)
  Time_Mark : Inport
  Enable : EnablePort
  Constant1 : Constant  Priority=28  OutDataTypeStr=boolean
  Constant2 : Constant  Priority=28  OutDataTypeStr=boolean
  Constant3 : Constant  Priority=24  OutDataTypeStr=boolean
  Constant4 : Constant  Value=0
  Data Store Read1 : DataStoreRead  Priority=11  DataStoreName=Desync_Ticks  IndexOptions=Index vector (dialog)  Indices=1  OutputSizes=1
  Data Store Write : DataStoreWrite  DataStoreName=Desync_Positive  IndexOptions=Index vector (dialog)  Indices=1  OutputSizes=1
  Data Store Write1 : DataStoreWrite  Priority=29  DataStoreName=Toggle_Pin_D10  IndexOptions=Index vector (dialog)  Indices=1  OutputSizes=1
  Data Store Write13 : DataStoreWrite  Priority=25  DataStoreName=BC1_Sync_processed  IndexOptions=Index vector (dialog)  Indices=1  OutputSizes=1
  Data Store Write3 : DataStoreWrite  Priority=29  DataStoreName=Toggle_Pin_A0  IndexOptions=Index vector (dialog)  Indices=1  OutputSizes=1
  Desync_Negative : Subsystem  TreatAsAtomicUnit=on
  GreaterThan : RelationalOperator  Operator=>  OutDataTypeStr=boolean  RndMeth=Simplest  InputSameDT=off
  NOT : Logic  Operator=NOT  IconShape=distinctive  AllPortsSameDT=off  OutDataTypeStr=boolean
  wires:
  Constant1/1 -> Data Store Write3/1
  Constant3/1 -> Data Store Write13/1
  Data Store Read1/1 -> GreaterThan/1
  Constant4/1 -> GreaterThan/2
  NOT/1 -> Desync_Negative/Enable
  GreaterThan/1 -> NOT/1, Data Store Write/1
  Time_Mark/1 -> Desync_Negative/1(Current_Local_Time)
  Constant2/1 -> Data Store Write1/1

== system HANcoder_E407_TTA_Template_DS_V52/HANcoder STM32 Target - E407-STM32 algorithm/TTA CAN System/TTA System/Matrix Cycle Manager/Controller Matrix Cycle/controller basic cycle 2/COMM Task - Articualtion angle trailer 1/Reception substasks ==
  note: Still no msg received
  note: Beginning of the task
  note: LT == TM_COMM
  note: LT > TM_COMM
  note: After the beginning of the task
  Time_Mark : Inport
  RX_ID : Inport  Port=2
  Enable : EnablePort
  AND : Logic  IconShape=distinctive  AllPortsSameDT=off  OutDataTypeStr=boolean
  AND1 : Logic  IconShape=distinctive  AllPortsSameDT=off  OutDataTypeStr=boolean
  Data Store Read : DataStoreRead  DataStoreName=Local_Ticks  IndexOptions=Index vector (dialog)  Indices=1  OutputSizes=1
  Data Store Read1 : DataStoreRead  DataStoreName=New_Msg_Ready_CAN1  IndexOptions=Index vector (dialog)  Indices=1  OutputSizes=1
  Data Store Read2 : DataStoreRead  DataStoreName=New_Msg_Ready_CAN2  IndexOptions=Index vector (dialog)  Indices=1  OutputSizes=1
  Equal16 : RelationalOperator  Operator===  OutDataTypeStr=boolean  RndMeth=Simplest  InputSameDT=off
  Equal2 : RelationalOperator  Operator=>  OutDataTypeStr=boolean  RndMeth=Simplest  InputSameDT=off
  NOT : Logic  Operator=NOT  IconShape=distinctive  AllPortsSameDT=off  OutDataTypeStr=boolean
  NOT1 : Logic  Operator=NOT  IconShape=distinctive  AllPortsSameDT=off  OutDataTypeStr=boolean
  RX buffers update : Subsystem  Priority=20
  Receive CAN1 : Outport  OutputWhenDisabled=reset  InitialOutput=0  VectorParamsAs1DForOutWhenUnconnected=off
  Receive CAN2 : Outport  Port=2  OutputWhenDisabled=reset  InitialOutput=0  VectorParamsAs1DForOutWhenUnconnected=off
  wires:
  Time_Mark/1 -> Equal2/2, Equal16/2
  Data Store Read/1 -> Equal2/1, Equal16/1
  Equal16/1 -> RX buffers update/Enable
  RX_ID/1 -> RX buffers update/1(Rx_ID)
  Data Store Read1/1 -> NOT/1
  Data Store Read2/1 -> NOT1/1
  NOT1/1 -> AND1/2
  NOT/1 -> AND/2
  Equal2/1 -> AND1/1, AND/1
  AND/1 -> Receive CAN1/1
  AND1/1 -> Receive CAN2/1

== system HANcoder_E407_TTA_Template_DS_V52/HANcoder STM32 Target - E407-STM32 algorithm/TTA CAN System/TTA System/Matrix Cycle Manager/Controller Matrix Cycle/controller basic cycle 2/COMM Task - Articualtion angle trailer 1/Transmission subtasks ==
  note: Encode value domain message at the start of the task
  note: Beginning of the task
  note: LT == TM_COMM
  note: LT > TM_COMM
  note: After the beginning of the task
  note: Check if we have not surpassed
      | maximum number of Tx messages
  note: Check if we have not surpassed
      | maximum number of Tx messages
  Time_Mark : Inport
  TX_ID : Inport  Port=2
  Enable : EnablePort
  AND : Logic  IconShape=distinctive  AllPortsSameDT=off  OutDataTypeStr=boolean
  AND1 : Logic  IconShape=distinctive  AllPortsSameDT=off  OutDataTypeStr=boolean
  Check msg transmission CAN1 : Subsystem
  Check msg transmission CAN2 : Subsystem
  Constant6 : Constant  Value=max_num_msgs_CAN1
  Constant7 : Constant  Value=max_num_msgs_CAN2
  Data Store Read : DataStoreRead  DataStoreName=Local_Ticks  IndexOptions=Index vector (dialog)  Indices=1  OutputSizes=1
  Data Store Read2 : DataStoreRead  DataStoreName=Tx_msg_count_CAN1  IndexOptions=Index vector (dialog)  Indices=1  OutputSizes=1
  Data Store Read3 : DataStoreRead  DataStoreName=Tx_msg_count_CAN2  IndexOptions=Index vector (dialog)  Indices=1  OutputSizes=1
  Equal16 : RelationalOperator  Operator===  OutDataTypeStr=boolean  RndMeth=Simplest  InputSameDT=off
  Equal2 : RelationalOperator  Operator=>  OutDataTypeStr=boolean  RndMeth=Simplest  InputSameDT=off
  GreaterThan2 : RelationalOperator  Operator=<=  OutDataTypeStr=boolean  RndMeth=Simplest  InputSameDT=off
  GreaterThan3 : RelationalOperator  Operator=<=  OutDataTypeStr=boolean  RndMeth=Simplest  InputSameDT=off
  Msg_Value_Data_Encoded : Subsystem
  Send CAN1 : Outport  OutputWhenDisabled=reset  InitialOutput=0  VectorParamsAs1DForOutWhenUnconnected=off
  Send CAN2 : Outport  Port=2  OutputWhenDisabled=reset  InitialOutput=0  VectorParamsAs1DForOutWhenUnconnected=off
  wires:
  Time_Mark/1 -> Check msg transmission CAN1/2(Time Mark), Check msg transmission CAN2/2(Time Mark), Equal2/2, Equal16/2
  Data Store Read/1 -> Check msg transmission CAN1/1(Local Time), Check msg transmission CAN2/1(Local Time), Equal2/1, Equal16/1
  Equal16/1 -> Msg_Value_Data_Encoded/Enable
  Check msg transmission CAN1/1(Send CAN1) -> Send CAN1/1
  Check msg transmission CAN2/1(Send CAN2) -> Send CAN2/1
  Data Store Read2/1 -> GreaterThan2/1
  Constant6/1 -> GreaterThan2/2
  Constant7/1 -> GreaterThan3/2
  Data Store Read3/1 -> GreaterThan3/1
  GreaterThan2/1 -> AND/2
  AND/1 -> Check msg transmission CAN1/Enable
  AND1/1 -> Check msg transmission CAN2/Enable
  GreaterThan3/1 -> AND1/2
  Msg_Value_Data_Encoded/1(Value_domain_msg) -> [Encoded_msg_TAG]
  [Encoded_msg_TAG] -> Check msg transmission CAN1/4(Value Domain Msg)
  [Encoded_msg_TAG] -> Check msg transmission CAN2/4(Value Domain Msg)
  TX_ID/1 -> [Tx_ID_TAG]
  [Tx_ID_TAG] -> Check msg transmission CAN1/3(Tx_ID)
  [Tx_ID_TAG] -> Check msg transmission CAN2/3(Tx_ID)
  Equal2/1 -> [Next_actions_TAG]
  [Next_actions_TAG] -> AND/1
  [Next_actions_TAG] -> AND1/1

== system HANcoder_E407_TTA_Template_DS_V52/HANcoder STM32 Target - E407-STM32 algorithm/TTA CAN System/TTA System/Matrix Cycle Manager/Controller Matrix Cycle/controller basic cycle 2/COMM Task - Articualtion angle trailer 2/Reception substasks ==
  note: Still no msg received
  note: Beginning of the task
  note: LT == TM_COMM
  note: LT > TM_COMM
  note: After the beginning of the task
  Time_Mark : Inport
  RX_ID : Inport  Port=2
  Enable : EnablePort
  AND : Logic  IconShape=distinctive  AllPortsSameDT=off  OutDataTypeStr=boolean
  AND1 : Logic  IconShape=distinctive  AllPortsSameDT=off  OutDataTypeStr=boolean
  Data Store Read : DataStoreRead  DataStoreName=Local_Ticks  IndexOptions=Index vector (dialog)  Indices=1  OutputSizes=1
  Data Store Read1 : DataStoreRead  DataStoreName=New_Msg_Ready_CAN1  IndexOptions=Index vector (dialog)  Indices=1  OutputSizes=1
  Data Store Read2 : DataStoreRead  DataStoreName=New_Msg_Ready_CAN2  IndexOptions=Index vector (dialog)  Indices=1  OutputSizes=1
  Equal16 : RelationalOperator  Operator===  OutDataTypeStr=boolean  RndMeth=Simplest  InputSameDT=off
  Equal2 : RelationalOperator  Operator=>  OutDataTypeStr=boolean  RndMeth=Simplest  InputSameDT=off
  NOT : Logic  Operator=NOT  IconShape=distinctive  AllPortsSameDT=off  OutDataTypeStr=boolean
  NOT1 : Logic  Operator=NOT  IconShape=distinctive  AllPortsSameDT=off  OutDataTypeStr=boolean
  RX buffers update : Subsystem  Priority=20
  Receive CAN1 : Outport  OutputWhenDisabled=reset  InitialOutput=0  VectorParamsAs1DForOutWhenUnconnected=off
  Receive CAN2 : Outport  Port=2  OutputWhenDisabled=reset  InitialOutput=0  VectorParamsAs1DForOutWhenUnconnected=off
  wires:
  Time_Mark/1 -> Equal2/2, Equal16/2
  Data Store Read/1 -> Equal2/1, Equal16/1
  Equal16/1 -> RX buffers update/Enable
  RX_ID/1 -> RX buffers update/1(Rx_ID)
  Data Store Read1/1 -> NOT/1
  Data Store Read2/1 -> NOT1/1
  NOT1/1 -> AND1/2
  NOT/1 -> AND/2
  Equal2/1 -> AND1/1, AND/1
  AND/1 -> Receive CAN1/1
  AND1/1 -> Receive CAN2/1

== system HANcoder_E407_TTA_Template_DS_V52/HANcoder STM32 Target - E407-STM32 algorithm/TTA CAN System/TTA System/Matrix Cycle Manager/Controller Matrix Cycle/controller basic cycle 2/COMM Task - Articualtion angle trailer 2/Transmission subtasks ==
  note: Encode value domain message at the start of the task
  note: Beginning of the task
  note: LT == TM_COMM
  note: LT > TM_COMM
  note: After the beginning of the task
  note: Check if we have not surpassed
      | maximum number of Tx messages
  note: Check if we have not surpassed
      | maximum number of Tx messages
  Time_Mark : Inport
  TX_ID : Inport  Port=2
  Enable : EnablePort
  AND : Logic  IconShape=distinctive  AllPortsSameDT=off  OutDataTypeStr=boolean
  AND1 : Logic  IconShape=distinctive  AllPortsSameDT=off  OutDataTypeStr=boolean
  Check msg transmission CAN1 : Subsystem
  Check msg transmission CAN2 : Subsystem
  Constant6 : Constant  Value=max_num_msgs_CAN1
  Constant7 : Constant  Value=max_num_msgs_CAN2
  Data Store Read : DataStoreRead  DataStoreName=Local_Ticks  IndexOptions=Index vector (dialog)  Indices=1  OutputSizes=1
  Data Store Read2 : DataStoreRead  DataStoreName=Tx_msg_count_CAN1  IndexOptions=Index vector (dialog)  Indices=1  OutputSizes=1
  Data Store Read3 : DataStoreRead  DataStoreName=Tx_msg_count_CAN2  IndexOptions=Index vector (dialog)  Indices=1  OutputSizes=1
  Equal16 : RelationalOperator  Operator===  OutDataTypeStr=boolean  RndMeth=Simplest  InputSameDT=off
  Equal2 : RelationalOperator  Operator=>  OutDataTypeStr=boolean  RndMeth=Simplest  InputSameDT=off
  GreaterThan2 : RelationalOperator  Operator=<=  OutDataTypeStr=boolean  RndMeth=Simplest  InputSameDT=off
  GreaterThan3 : RelationalOperator  Operator=<=  OutDataTypeStr=boolean  RndMeth=Simplest  InputSameDT=off
  Msg_Value_Data_Encoded : Subsystem
  Send CAN1 : Outport  OutputWhenDisabled=reset  InitialOutput=0  VectorParamsAs1DForOutWhenUnconnected=off
  Send CAN2 : Outport  Port=2  OutputWhenDisabled=reset  InitialOutput=0  VectorParamsAs1DForOutWhenUnconnected=off
  wires:
  Time_Mark/1 -> Check msg transmission CAN1/2(Time Mark), Check msg transmission CAN2/2(Time Mark), Equal2/2, Equal16/2
  Data Store Read/1 -> Check msg transmission CAN1/1(Local Time), Check msg transmission CAN2/1(Local Time), Equal2/1, Equal16/1
  Equal16/1 -> Msg_Value_Data_Encoded/Enable
  Check msg transmission CAN1/1(Send CAN1) -> Send CAN1/1
  Check msg transmission CAN2/1(Send CAN2) -> Send CAN2/1
  Data Store Read2/1 -> GreaterThan2/1
  Constant6/1 -> GreaterThan2/2
  Constant7/1 -> GreaterThan3/2
  Data Store Read3/1 -> GreaterThan3/1
  GreaterThan2/1 -> AND/2
  AND/1 -> Check msg transmission CAN1/Enable
  AND1/1 -> Check msg transmission CAN2/Enable
  GreaterThan3/1 -> AND1/2
  Msg_Value_Data_Encoded/1(Value_domain_msg) -> [Encoded_msg_TAG]
  [Encoded_msg_TAG] -> Check msg transmission CAN1/4(Value Domain Msg)
  [Encoded_msg_TAG] -> Check msg transmission CAN2/4(Value Domain Msg)
  TX_ID/1 -> [Tx_ID_TAG]
  [Tx_ID_TAG] -> Check msg transmission CAN1/3(Tx_ID)
  [Tx_ID_TAG] -> Check msg transmission CAN2/3(Tx_ID)
  Equal2/1 -> [Next_actions_TAG]
  [Next_actions_TAG] -> AND/1
  [Next_actions_TAG] -> AND1/1

== system HANcoder_E407_TTA_Template_DS_V52/HANcoder STM32 Target - E407-STM32 algorithm/TTA CAN System/TTA System/Matrix Cycle Manager/Controller Matrix Cycle/controller basic cycle 2/COMM Task - Sync bc 1/Reception substasks ==
  note: Still no msg received
  note: Beginning of the task
  note: LT == TM_COMM
  note: LT > TM_COMM
  note: After the beginning of the task
  Time_Mark : Inport
  RX_ID : Inport  Port=2
  Enable : EnablePort
  AND : Logic  IconShape=distinctive  AllPortsSameDT=off  OutDataTypeStr=boolean
  AND1 : Logic  IconShape=distinctive  AllPortsSameDT=off  OutDataTypeStr=boolean
  Data Store Read : DataStoreRead  DataStoreName=Local_Ticks  IndexOptions=Index vector (dialog)  Indices=1  OutputSizes=1
  Data Store Read1 : DataStoreRead  DataStoreName=New_Msg_Ready_CAN1  IndexOptions=Index vector (dialog)  Indices=1  OutputSizes=1
  Data Store Read2 : DataStoreRead  DataStoreName=New_Msg_Ready_CAN2  IndexOptions=Index vector (dialog)  Indices=1  OutputSizes=1
  Equal16 : RelationalOperator  Operator===  OutDataTypeStr=boolean  RndMeth=Simplest  InputSameDT=off
  Equal2 : RelationalOperator  Operator=>  OutDataTypeStr=boolean  RndMeth=Simplest  InputSameDT=off
  NOT : Logic  Operator=NOT  IconShape=distinctive  AllPortsSameDT=off  OutDataTypeStr=boolean
  NOT1 : Logic  Operator=NOT  IconShape=distinctive  AllPortsSameDT=off  OutDataTypeStr=boolean
  RX buffers update : Subsystem  Priority=20
  Receive CAN1 : Outport  OutputWhenDisabled=reset  InitialOutput=0  VectorParamsAs1DForOutWhenUnconnected=off
  Receive CAN2 : Outport  Port=2  OutputWhenDisabled=reset  InitialOutput=0  VectorParamsAs1DForOutWhenUnconnected=off
  wires:
  Time_Mark/1 -> Equal2/2, Equal16/2
  Data Store Read/1 -> Equal2/1, Equal16/1
  Equal16/1 -> RX buffers update/Enable
  RX_ID/1 -> RX buffers update/1(Rx_ID)
  Data Store Read1/1 -> NOT/1
  Data Store Read2/1 -> NOT1/1
  NOT1/1 -> AND1/2
  NOT/1 -> AND/2
  Equal2/1 -> AND1/1, AND/1
  AND/1 -> Receive CAN1/1
  AND1/1 -> Receive CAN2/1

== system HANcoder_E407_TTA_Template_DS_V52/HANcoder STM32 Target - E407-STM32 algorithm/TTA CAN System/TTA System/Matrix Cycle Manager/Controller Matrix Cycle/controller basic cycle 2/COMM Task - Sync bc 1/Transmission subtasks1 ==
  note: Encode value domain message at the start of the task
  note: Beginning of the task
  note: LT == TM_COMM
  note: LT > TM_COMM
  note: After the beginning of the task
  note: Check if we have not surpassed
      | maximum number of Tx messages
  note: Check if we have not surpassed
      | maximum number of Tx messages
  Time_Mark : Inport
  TX_ID : Inport  Port=2
  Enable : EnablePort
  AND : Logic  IconShape=distinctive  AllPortsSameDT=off  OutDataTypeStr=boolean
  AND1 : Logic  IconShape=distinctive  AllPortsSameDT=off  OutDataTypeStr=boolean
  Check msg transmission CAN1 : Subsystem
  Check msg transmission CAN2 : Subsystem
  Constant6 : Constant  Value=max_num_msgs_CAN1
  Constant7 : Constant  Value=max_num_msgs_CAN2
  Data Store Read : DataStoreRead  DataStoreName=Local_Ticks  IndexOptions=Index vector (dialog)  Indices=1  OutputSizes=1
  Data Store Read2 : DataStoreRead  DataStoreName=Tx_msg_count_CAN1  IndexOptions=Index vector (dialog)  Indices=1  OutputSizes=1
  Data Store Read3 : DataStoreRead  DataStoreName=Tx_msg_count_CAN2  IndexOptions=Index vector (dialog)  Indices=1  OutputSizes=1
  Equal16 : RelationalOperator  Operator===  OutDataTypeStr=boolean  RndMeth=Simplest  InputSameDT=off
  Equal2 : RelationalOperator  Operator=>  OutDataTypeStr=boolean  RndMeth=Simplest  InputSameDT=off
  GreaterThan2 : RelationalOperator  Operator=<=  OutDataTypeStr=boolean  RndMeth=Simplest  InputSameDT=off
  GreaterThan3 : RelationalOperator  Operator=<=  OutDataTypeStr=boolean  RndMeth=Simplest  InputSameDT=off
  Msg_Value_Data_Encoded : Subsystem
  Send CAN1 : Outport  OutputWhenDisabled=reset  InitialOutput=0  VectorParamsAs1DForOutWhenUnconnected=off
  Send CAN2 : Outport  Port=2  OutputWhenDisabled=reset  InitialOutput=0  VectorParamsAs1DForOutWhenUnconnected=off
  wires:
  Time_Mark/1 -> Check msg transmission CAN1/2(Time Mark), Check msg transmission CAN2/2(Time Mark), Equal2/2, Equal16/2
  Data Store Read/1 -> Check msg transmission CAN1/1(Local Time), Check msg transmission CAN2/1(Local Time), Equal2/1, Equal16/1
  Equal16/1 -> Msg_Value_Data_Encoded/Enable
  Check msg transmission CAN1/1(Send CAN1) -> Send CAN1/1
  Check msg transmission CAN2/1(Send CAN2) -> Send CAN2/1
  Data Store Read2/1 -> GreaterThan2/1
  Constant6/1 -> GreaterThan2/2
  Constant7/1 -> GreaterThan3/2
  Data Store Read3/1 -> GreaterThan3/1
  GreaterThan2/1 -> AND/2
  AND/1 -> Check msg transmission CAN1/Enable
  AND1/1 -> Check msg transmission CAN2/Enable
  GreaterThan3/1 -> AND1/2
  Msg_Value_Data_Encoded/1(Value_domain_msg) -> [Encoded_msg_TAG]
  [Encoded_msg_TAG] -> Check msg transmission CAN1/4(Value Domain Msg)
  [Encoded_msg_TAG] -> Check msg transmission CAN2/4(Value Domain Msg)
  TX_ID/1 -> [Tx_ID_TAG]
  [Tx_ID_TAG] -> Check msg transmission CAN1/3(Tx_ID)
  [Tx_ID_TAG] -> Check msg transmission CAN2/3(Tx_ID)
  Equal2/1 -> [Next_actions_TAG]
  [Next_actions_TAG] -> AND/1
  [Next_actions_TAG] -> AND1/1
